simulink model "twobus_transient_sim_explicit"  (R2020b)
settings: Solver=VariableStepAuto  StartTime=0.0  StopTime=1  RelTol=1e-3
libraries: powerlib x38
settings Model: Creator=tmcnama2  LastModifiedBy=tmcnama2

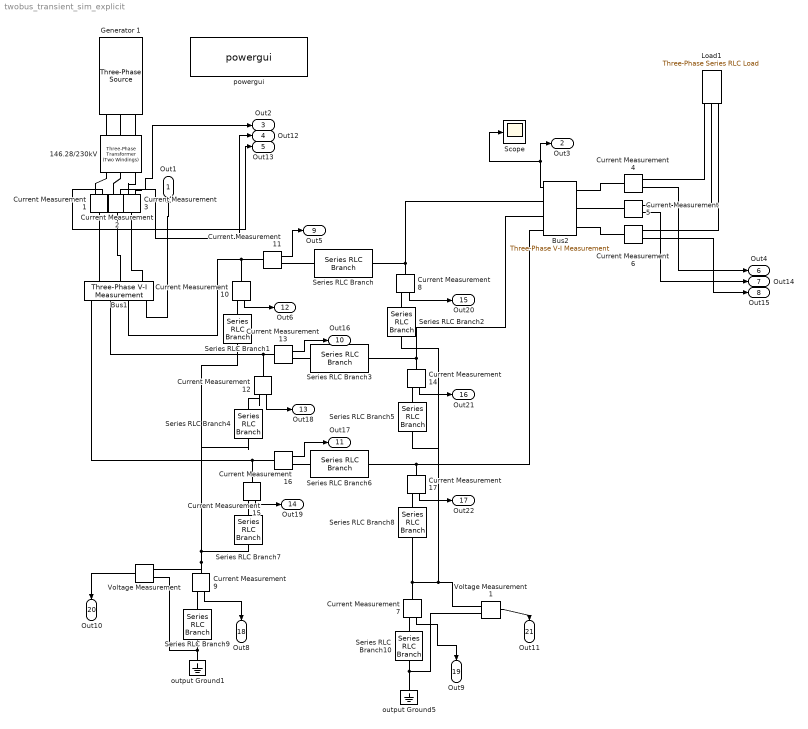
== system twobus_transient_sim_explicit ==
  146.28/230kV : powerlib/Elements/Three-Phase Transformer (Two Windings)  Winding1Connection=Yg  Winding2Connection=Yg  CoreType=Three single-phase transformers  SetSaturation=off  Hysteresis=off  DataFile='hysteresis'  SetInitialFlux=off  Measurements=None  UNITS=pu  NominalPower=[ 120e6 , 60 ]  Winding1=[146.28e3 , 0.002 , 0.08 ]  Winding2=[ 230e3 , 0.002 , 0.08 ]  Rm=500  Lm=500  L0=0.5  Saturation=[ 0,0 ; 0.0024,1.2 ; 1.0,1.52 ]  InitialFluxes=[ 0.8 , -0.8 , 0.7 ]  BreakLoop=off  DiscreteSolver=Trapezoidal iterative  DataType=off  TransfoNumber=1
  Bus1 : powerlib/Measurements/Three-Phase V-I Measurement  VoltageMeasurement=phase-to-ground  SetLabelV=off  LabelV=VB1  Vpu=off  VpuLL=off  CurrentMeasurement=no  SetLabelI=off  LabelI=IB1  Ipu=off  Pbase=100e6  Vbase=500e3  OutputType=Complex  PhasorSimulation=off  PSBequivalent=0
  Bus2 : powerlib/Measurements/Three-Phase V-I Measurement  VoltageMeasurement=phase-to-ground  SetLabelV=off  LabelV=VB2  Vpu=off  VpuLL=off  CurrentMeasurement=no  SetLabelI=off  LabelI=IB2  Ipu=off  Pbase=100e6  Vbase=500e3  OutputType=Complex  PhasorSimulation=off  PSBequivalent=0
  Current Measurement{1..17} (17 alike) : powerlib/Measurements/Current Measurement  PhasorSimulation=off  OutputType=Complex  PSBequivalent=0
  Generator 1 : powerlib/Electrical Sources/Three-Phase Source  InternalConnection=Yg  VoltagePhases=off  Voltage=146280  PhaseAngle=0  Voltage_phases=[25e3 25e3 25e3]/sqrt(3)  PhaseAngles_phases=[0 -120 +120]  Frequency=60  NonIdealSource=on  SpecifyImpedance=off  Resistance=0.8929  Inductance=0.0166  ShortCircuitLevel=100e6  BaseVoltage=146.28e3  XRratio=7  BusType=PV  Pref=163e6  Qref=0  Prefabc=[10e3, 10e3, 10e3]  Qrefabc=[0, 0, 0]  Qmin=-inf  Qmax=inf
  Load1 : powerlib/Elements/Three-Phase Series RLC Load  LConnTagsString=A|B|C  Configuration=Y (grounded)  NominalVoltage=(230000)*0.941818  Vabc=[1e3 1e3 1e3]  Vabcp=[1e3 1e3 1e3]  NominalFrequency=60  UnbalancedPower=off  ActivePower=160e6  InductivePower=100e6  CapacitivePower=0  Pabc=[10e3 9e3 11e3]  QLabc=[100 90 110]  QCabc=[100 90 110]  Pabcp=[10e3 9e3 11e3]  QLabcp=[100 90 110]  QCabcp=[100 90 110]  Measurements=None  LoadType=constant PQ
  Scope : Scope
  Series RLC Branch : powerlib/Elements/Series RLC Branch  LConnTagsString=__new0  RConnTagsString=__new0  BranchType=RL  Resistance=1.2730  Inductance=0.41264  SetiL0=off  InitialCurrent=0  Capacitance=1e-6  Setx0=off  InitialVoltage=0  Measurements=None
  Series RLC Branch{1..2,4..5,7..8} (6 alike) : powerlib/Elements/Series RLC Branch  LConnTagsString=__new0  RConnTagsString=__new0  BranchType=C  Resistance=1.2730  Inductance=0.4126  SetiL0=off  InitialCurrent=0  Capacitance=1.2740e-06/2  Setx0=off  InitialVoltage=0  Measurements=None
  Series RLC Branch10 : powerlib/Elements/Series RLC Branch  LConnTagsString=__new0  RConnTagsString=__new0  BranchType=C  Resistance=1.2730  Inductance=0.4126  SetiL0=off  InitialCurrent=0  Capacitance=5.9360e-06/2  Setx0=off  InitialVoltage=0  Measurements=None
  Series RLC Branch3 : powerlib/Elements/Series RLC Branch  LConnTagsString=__new0  RConnTagsString=__new0  BranchType=RL  Resistance=1.2730  Inductance=0.41264  SetiL0=off  InitialCurrent=0  Capacitance=1e-6  Setx0=off  InitialVoltage=0  Measurements=None
  Series RLC Branch6 : powerlib/Elements/Series RLC Branch  LConnTagsString=__new0  RConnTagsString=__new0  BranchType=RL  Resistance=1.2730  Inductance=0.41264  SetiL0=off  InitialCurrent=0  Capacitance=1e-6  Setx0=off  InitialVoltage=0  Measurements=None
  Series RLC Branch9 : powerlib/Elements/Series RLC Branch  LConnTagsString=__new0  RConnTagsString=__new0  BranchType=C  Resistance=1.2730  Inductance=0.4126  SetiL0=off  InitialCurrent=0  Capacitance=5.9360e-06/2  Setx0=off  InitialVoltage=0  Measurements=None
  Voltage Measurement : powerlib/Measurements/Voltage Measurement  PhasorSimulation=off  OutputType=Complex  PSBequivalent=0
  Voltage Measurement1 : powerlib/Measurements/Voltage Measurement  PhasorSimulation=off  OutputType=Complex  PSBequivalent=0
  output Ground1 : powerlib/Elements/Ground  LConnTagsString=a
  output Ground5 : powerlib/Elements/Ground  LConnTagsString=a
  powergui : powerlib/powergui  Priority=1  SimulationMode=Discrete  SampleTime=50e-6  frequency=60  Iterations=50  frequencyindice=60  Pbase=120e6  ErrMax=0.0001  UnitsV=kV  UnitsW=MW  buscounter=0  FunctionMessages=off  echomessages=off  EnableUseOfTLC=off  CurrentSourceSwitches=off  DisableSnubberDevices=off  DisableRonSwitches=off  DisableVfSwitches=off  DisplayEquations=off  AutomaticDiscreteSolvers=off  SolverType=Tustin/Backward Euler (TBE)  Interpol=off  ExternalGateDelay=off  methode=off  Ts=100  x0status=zero  SPID=on  SwTol=0  HookPort=off  NonlinearTolerance=1e-4  nMaxIteration=100  ContinueOnMaxIteration=off  RestoreLinks=warning  ResistiveCurrentMeasurement=off  Frange=[0:2:500]  Ylog=off  Xlog=on  ShowGrid=off  save=off  variable=ZData  structure=0  ZoomFFT=off  StartTime=0.0  cycles=1  DisplayStyle=1  fundamental=60  FreqAxis=off  MaxFrequency=1000  frequencyindicesteady=1  RmsSteady=1  display=off
  Out1 : Outport  SignalName=V1
  Out3 : Outport  Port=2  SignalName=V2
  Out2 : Outport  Port=3  SignalName=I1a
  Out12 : Outport  Port=4  SignalName=I1b
  Out13 : Outport  Port=5  SignalName=I1c
  Out4 : Outport  Port=6  SignalName=I2a
  Out14 : Outport  Port=7  SignalName=I2b
  Out15 : Outport  Port=8  SignalName=I2c
  Out5 : Outport  Port=9  SignalName=Ib_series_a
  Out16 : Outport  Port=10  SignalName=Ib_series_b
  Out17 : Outport  Port=11  SignalName=Ib_series_c
  Out6 : Outport  Port=12  SignalName=Ib_csh_fr_a
  Out18 : Outport  Port=13  SignalName=Ib_csh_fr_b
  Out19 : Outport  Port=14  SignalName=Ib_csh_fr_c
  Out20 : Outport  Port=15  SignalName=Ib_csh_to_a
  Out21 : Outport  Port=16  SignalName=Ib_csh_to_b
  Out22 : Outport  Port=17  SignalName=Ib_csh_to_c
  Out8 : Outport  Port=18  SignalName=Ib_cg_fr
  Out9 : Outport  Port=19  SignalName=Ib_cgnd_to
  Out10 : Outport  Port=20  SignalName=Vn_cg_fr
  Out11 : Outport  Port=21  SignalName=Vn_cg_fr
  wires:
  Bus2/1 -> Scope/1, Out3/1
  Current Measurement3/1 -> Out2/1
  Current Measurement2/1 -> Out12/1
  Current Measurement1/1 -> Out13/1
  Current Measurement11/1 -> Out5/1
  Current Measurement13/1 -> Out16/1
  Current Measurement16/1 -> Out17/1
  Current Measurement12/1 -> Out18/1
  Current Measurement14/1 -> Out21/1
  Current Measurement9/1 -> Out8/1
  Current Measurement7/1 -> Out9/1
  Voltage Measurement1/1 -> Out11/1
  Voltage Measurement/1 -> Out10/1
  Bus1/1 -> Out1/1
  Current Measurement8/1 -> Out20/1
  Current Measurement17/1 -> Out22/1
  Current Measurement10/1 -> Out6/1
  Current Measurement15/1 -> Out19/1
  Current Measurement4/1 -> Out4/1
  Current Measurement5/1 -> Out14/1
  Current Measurement6/1 -> Out15/1
  connections:
  Generator 1/RConn3 -- 146.28/230kV/LConn3
  Generator 1/RConn2 -- 146.28/230kV/LConn2
  146.28/230kV/LConn1 -- Generator 1/RConn1
  Current Measurement4/RConn1 -- Load1/LConn1
  Current Measurement5/RConn1 -- Load1/LConn2
  Current Measurement6/RConn1 -- Load1/LConn3
  Current Measurement4/LConn1 -- Bus2/LConn1
  Current Measurement5/LConn1 -- Bus2/LConn2
  Current Measurement6/LConn1 -- Bus2/LConn3
  output Ground5/LConn1 -- Voltage Measurement1/LConn2 -- Series RLC Branch10/RConn1
  output Ground1/LConn1 -- Voltage Measurement/LConn2 -- Series RLC Branch9/RConn1
  Current Measurement8/RConn1 -- Series RLC Branch2/LConn1
  Series RLC Branch/RConn1 -- Bus2/RConn1 -- Current Measurement8/LConn1
  Current Measurement7/RConn1 -- Series RLC Branch10/LConn1
  Current Measurement9/RConn1 -- Series RLC Branch9/LConn1
  Current Measurement10/RConn1 -- Series RLC Branch1/LConn1
  Current Measurement11/RConn1 -- Series RLC Branch/LConn1
  Current Measurement10/LConn1 -- Bus1/RConn1 -- Current Measurement11/LConn1
  Current Measurement12/LConn1 -- Bus1/RConn2 -- Current Measurement13/LConn1
  Current Measurement12/RConn1 -- Series RLC Branch4/LConn1
  Current Measurement13/RConn1 -- Series RLC Branch3/LConn1
  Series RLC Branch3/RConn1 -- Bus2/RConn2 -- Current Measurement14/LConn1
  Current Measurement14/RConn1 -- Series RLC Branch5/LConn1
  Current Measurement15/LConn1 -- Bus1/RConn3 -- Current Measurement16/LConn1
  Current Measurement15/RConn1 -- Series RLC Branch7/LConn1
  Current Measurement16/RConn1 -- Series RLC Branch6/LConn1
  Series RLC Branch6/RConn1 -- Bus2/RConn3 -- Current Measurement17/LConn1
  Current Measurement17/RConn1 -- Series RLC Branch8/LConn1
  Current Measurement9/LConn1 -- Series RLC Branch4/RConn1 -- Series RLC Branch1/RConn1 -- Series RLC Branch7/RConn1 -- Voltage Measurement/LConn1
  Current Measurement7/LConn1 -- Voltage Measurement1/LConn1 -- Series RLC Branch2/RConn1 -- Series RLC Branch5/RConn1 -- Series RLC Branch8/RConn1
  Current Measurement3/RConn1 -- 146.28/230kV/RConn1
  Bus1/LConn1 -- Current Measurement3/LConn1
  Current Measurement2/RConn1 -- 146.28/230kV/RConn2
  Bus1/LConn2 -- Current Measurement2/LConn1
  Current Measurement1/RConn1 -- 146.28/230kV/RConn3
  Current Measurement1/LConn1 -- Bus1/LConn3
